simulink model "ME295B_Controller1Sim"  (R2018b)
settings: Solver=ode5  StartTime=0.0  StopTime=15  FixedStep=0.0001  RelTol=1e-3  EnableMultiTasking=on
values from neighbouring files (symbols this model uses):
  amp = [pi/4 pi/8 pi/5]    [ME295B_Controller1.m]
  freq = [f f*2 f*3]    [ME295B_Controller1.m]
  Ka = 10.*diag(ones(1,length(Phi)))    [ME295B_Controller1.m]
  Lambda = (p/2).*diag(ones(1,3))    [ME295B_Controller1.m]
  Phi_hat_max = (1+BoundsRatio)*Phi_hat_o    [ME295B_Controller1.m]
  Phi_hat_min = (1-BoundsRatio)*Phi_hat_o    [ME295B_Controller1.m]
  Phi_hat_o = Phi.*z'    [ME295B_Controller1.m]
settings Model: Creator=Alan  LastModifiedBy=adeli
settings DataIOCC: LimitDataPoints=on  SaveFormat=Array
settings OptimizationCC: LifeSpan=inf
settings DebuggingCC: SFUnexpectedBacktrackingDiag=warning  SFNoUnconditionalDefaultTransitionDiag=warning  SFExecutionAtInitializationDiag=none
settings HardwareCC: ProdBitPerPointer=32  ProdBitPerSizeT=32  ProdBitPerPtrDiffT=32  ProdLargestAtomicFloat=None  ProdIntDivRoundTo=Undefined  ProdEndianess=Unspecified  ProdWordSize=32  ProdHWDeviceType=32-bit Generic
settings ModelReferenceCC: PropagateSignalLabelsOutOfModel=off
settings SFSimCC: SimUseLocalCustomCode=off
settings RTWCC: RTWUseLocalCustomCode=off
settings CodeAppCC: StateflowObjectComments=on
settings GRTTargetCC: TargetLangStandard=C89/C90 (ANSI)  GeneratePreprocessorConditionals=Disable all
settings ConfigComp: CovMetricSettings=dw  CovHtmlReporting=on  CovSaveCumulativeToWorkspaceVar=on  CovSaveSingleToWorkspaceVar=on  CovExternalEMLEnable=off

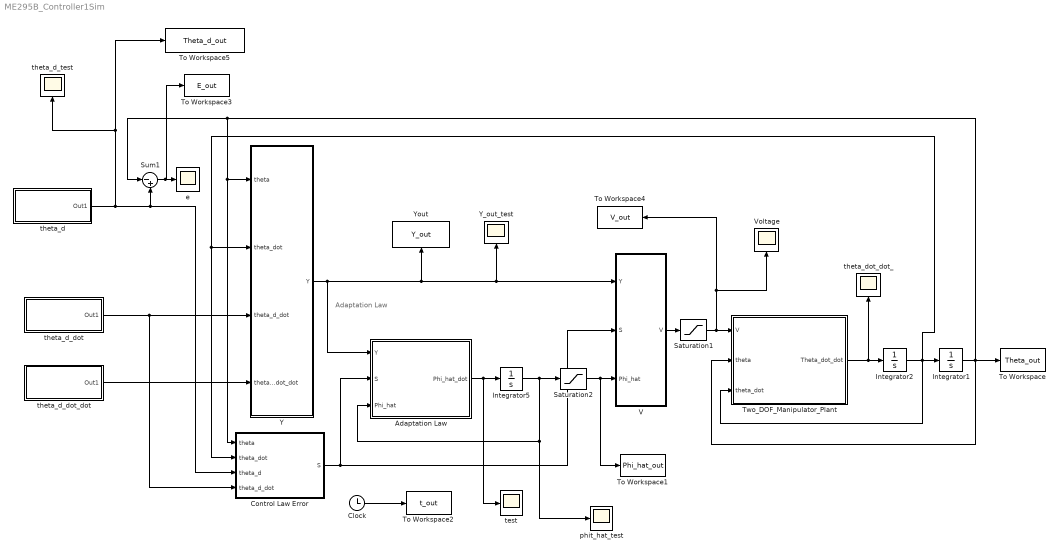
== system ME295B_Controller1Sim ==
  note: Adaptation Law
  Adaptation Law : MATLAB Function  TreatAsAtomicUnit=on
  Clock : Clock
  Control Law Error : MATLAB Function  TreatAsAtomicUnit=on
  Integrator1 : Integrator  InitialCondition=[0;0;0]
  Integrator2 : Integrator  InitialCondition=[0;0;0]
  Integrator5 : Integrator  InitialCondition=Phi_hat_o
  Saturation1 : Saturate  UpperLimit=[24, 24, 24]  LowerLimit=[-24, -24, -24]
  Saturation2 : Saturate  UpperLimit=1000000  LowerLimit=0
  Sum1 : Sum  Inputs=|-+
  To Workspace : ToWorkspace  VariableName=Theta_out  SampleTime=-1
  To Workspace1 : ToWorkspace  VariableName=Phi_hat_out  SampleTime=-1
  To Workspace2 : ToWorkspace  VariableName=t_out  SampleTime=-1
  To Workspace3 : ToWorkspace  VariableName=E_out  SampleTime=-1
  To Workspace4 : ToWorkspace  VariableName=V_out  SampleTime=-1
  To Workspace5 : ToWorkspace  VariableName=Theta_d_out  SampleTime=-1
  Two_DOF_Manipulator_Plant : MATLAB Function  TreatAsAtomicUnit=on
  V : MATLAB Function  TreatAsAtomicUnit=on
  Voltage : Scope
  Y : MATLAB Function  TreatAsAtomicUnit=on
  Y_out_test : Scope
  Yout : ToWorkspace  VariableName=Y_out  SampleTime=-1
  e : Scope
  "phit_hat_test " : Scope
  test : Scope
  theta_d : Subsystem
  theta_d_dot : Subsystem
  theta_d_dot_dot : Subsystem
  theta_d_test : Scope
  theta_dot_dot_ : Scope
  wires:
  theta_d_dot_dot/1(Out1) -> Y/4(theta_d_dot_dot)
  Integrator2/1 -> Integrator1/1, Two_DOF_Manipulator_Plant/3(theta_dot), Control Law Error/2(theta_dot), Y/2(theta_dot)
  Integrator1/1 -> To Workspace/1, Two_DOF_Manipulator_Plant/2(theta), Control Law Error/1(theta), Y/1(theta), Sum1/1
  Sum1/1 -> To Workspace3/1, e/1
  Y/1(Y) -> Yout/1, Y_out_test/1, V/1(Y), Adaptation Law/1(Y)
  Control Law Error/1(S) -> V/2(S), Adaptation Law/2(S)
  Adaptation Law/1(Phi_hat_dot) -> Integrator5/1, test/1
  Integrator5/1 -> Saturation2/1, Adaptation Law/3(Phi_hat), "phit_hat_test "/1
  Two_DOF_Manipulator_Plant/1(Theta_dot_dot) -> theta_dot_dot_/1, Integrator2/1
  Clock/1 -> To Workspace2/1
  theta_d_dot/1(Out1) -> Control Law Error/4(theta_d_dot), Y/3(theta_d_dot)
  Saturation2/1 -> To Workspace1/1, V/3(Phi_hat)
  V/1(V) -> Saturation1/1
  Saturation1/1 -> Voltage/1, To Workspace4/1, Two_DOF_Manipulator_Plant/1(V)
  theta_d/1(Out1) -> theta_d_test/1, To Workspace5/1, Control Law Error/3(theta_d), Sum1/2

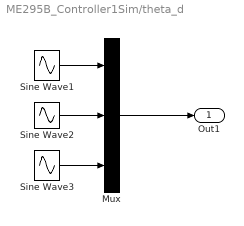
== system ME295B_Controller1Sim/theta_d ==
  Mux : Mux  Inputs=3
  Sine Wave1 : Sin  Amplitude=amp(1)  Frequency=freq(1)  SampleTime=0
  Sine Wave2 : Sin  Amplitude=amp(2)  Frequency=freq(2)  SampleTime=0
  Sine Wave3 : Sin  Amplitude=amp(1)  Frequency=freq(1)  SampleTime=0
  Out1 : Outport
  wires:
  Mux/1 -> Out1/1
  Sine Wave1/1 -> Mux/1
  Sine Wave2/1 -> Mux/2
  Sine Wave3/1 -> Mux/3

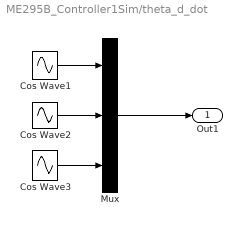
== system ME295B_Controller1Sim/theta_d_dot ==
  Cos Wave1 : Sin  Amplitude=freq(1)*amp(1)  Frequency=freq(1)  Phase=3.14/2  SampleTime=0
  Cos Wave2 : Sin  Amplitude=freq(2)*amp(2)  Frequency=freq(2)  Phase=3.14/2  SampleTime=0
  Cos Wave3 : Sin  Amplitude=freq(1)*amp(1)  Frequency=freq(1)  Phase=3.14/2  SampleTime=0
  Mux : Mux  Inputs=3
  Out1 : Outport
  wires:
  Mux/1 -> Out1/1
  Cos Wave1/1 -> Mux/1
  Cos Wave2/1 -> Mux/2
  Cos Wave3/1 -> Mux/3

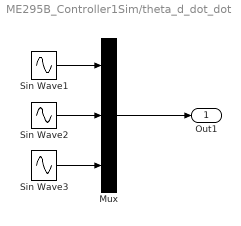
== system ME295B_Controller1Sim/theta_d_dot_dot ==
  Mux : Mux  Inputs=3
  Sin Wave1 : Sin  Amplitude=-freq(1)*freq(1)*amp(1)  Frequency=freq(1)  Phase=3.14/2  SampleTime=0
  Sin Wave2 : Sin  Amplitude=-freq(2)*freq(2)*amp(2)  Frequency=freq(2)  Phase=3.14/2  SampleTime=0
  Sin Wave3 : Sin  Amplitude=-freq(1)*freq(1)*amp(1)  Frequency=freq(1)  Phase=3.14/2  SampleTime=0
  Out1 : Outport
  wires:
  Mux/1 -> Out1/1
  Sin Wave1/1 -> Mux/1
  Sin Wave2/1 -> Mux/2
  Sin Wave3/1 -> Mux/3

== matlab function ME295B_Controller1Sim/V ==
  data: Eta parameter; V output; Y input; S input; Phi_hat input
function V = fcn(Eta, Y, S, Phi_hat)

V = (Y*Phi_hat) + Eta*S;

== matlab function ME295B_Controller1Sim/Y ==
  data: Lambda parameter; Y output; theta input; theta_dot input; theta_d_dot input; theta_d_dot_dot input; Phi_hat_o parameter
function Y = fcn(Lambda, theta, theta_dot,...
    theta_d_dot, theta_d_dot_dot, Phi_hat_o)

%errors and lambdas
e_dot1 = theta_d_dot(1,1)-theta_dot(1,1);
e_dot2 = theta_d_dot(2,1)-theta_dot(2,1);
e_dot3 = theta_d_dot(3,1)-theta_dot(3,1);

lambda1= Lambda(1,1);
lambda2 = Lambda(2,2);
lambda3 = Lambda(3,3);

theta_dot_dot1 = theta_d_dot_dot(1,1)+(lambda1*e_dot1);
theta_dot_dot2 = theta_d_dot_dot(2,1)+(lambda2*e_dot2);
theta_dot_dot3 = theta_d_dot_dot(3,1)+(lambda3*e_dot3);

%beta2 divided by beta1
k2_k1 = Phi_hat_o(2)/Phi_hat_o(1);
k3_k1 = Phi_hat_o(3)/Phi_hat_o(1);
k3_k2 = Phi_hat_o(3)/Phi_hat_o(2);

%first linkage
y11 = 2*( theta_dot_dot1*cos(theta(2,1)*cos(theta(2,1)+theta(3,1))) -...
    (theta_dot(1,1)*theta_dot(3,1)*cos(theta(2,1))*sin(theta(2,1)+theta(3,1))) -...
    (theta_dot(1,1)*theta_dot(2,1)*sin( (2*theta(2,1)) +theta(3,1))) );
y12=0;
y13=0;
y14 = 0;
y15 = (theta_dot_dot1)*(cos(theta(2,1))^2 ) +...
    -(2*theta_dot(1,1)*theta_dot(2,1)*sin(2*theta(2,1)));
y16 = (theta_dot_dot1)*(cos(theta(2,1)+theta(3,1)))^2 +...
    -2*theta_dot(1,1)*theta_dot(3,1)*cos(theta(2,1)+theta(3,1))*sin(theta(2,1)+theta(3,1)) +...
    -2*theta_dot(1,1)*theta_dot(2,1)*sin(2*(theta_dot(2,1)+theta(3,1)));
y17 = (sin(theta(2,1))^2)+...
    (2*theta_dot(1,1)*theta_dot(2,1)*sin(2*theta(2,1)));
y18 = (theta_dot_dot1)*(sin(theta(2,1)+theta(3,1))^2)+...
    2*theta_dot(1,1)*theta_dot(3,1)*cos(theta(2,1)+theta(3,1))*sin(theta(2,1)+theta(3,1)) +...
    2*theta_dot(1,1)*theta_dot(2,1)*sin(2*(theta_dot(2,1)+theta(3,1)));
y19 = theta_dot_dot1;
y110 = 0;
y111 = 0;
y112 = 0;
y113 = 0;
y114 = theta_dot(1,1);
y115 = 0;
y116 = 0;
%second linkage
y21 = 0;
y22 =2*theta_dot_dot2 +...
    theta_dot_dot3*cos(theta(3,1)) - ...
    theta_dot(3,1)*(theta_dot(2,1)+theta_dot(3,1)) -...
    (theta_dot(2,1)*theta_dot(3,1)*sin(theta(3,1))) +...
    (theta_dot(1,1)^2)*sin( (2*theta(2,1)) +theta(3,1));
y23 = 0;
y24 = -cos(theta(2,1))+...
    cos(theta(2,1)+theta(3,1));
y25 = k2_k1*(0.5*theta_dot(1,1)^2)*sin(2*theta(2,1));
y26 = k2_k1*(0.5*(theta_dot(1,1)^2)*sin(2*(theta(2,1)+theta(3,1))) );
y27 = k2_k1*(-0.5*theta_dot(1,1)^2)*sin(2*theta(2,1));
y28 = k2_k1*(-0.5*(theta_dot(1,1)^2)*sin(2*(theta(2,1)+theta(3,1))) );
y29 = 0;
y210 = sin(theta(2,1));
y211 =sin(theta(2,1)+theta(3,1));
y212= theta_dot_dot3;
y213=theta_dot_dot2;
y214=0;
y215=theta_dot(2,1);
y216=0;
%3rd linkage
y31 = 0;
y32 =0;
y33 = (theta_dot(1,1)^2)*cos(theta(2,1))*sin(theta(2,1)+theta(3,1)) +...
    theta_dot_dot2*cos(theta(3,1)) +...
    sin(theta(3,1));
y34 = 0;
y35 = 0;
y36 = k3_k1*(theta_dot(1,1)^2)*cos(theta(2,1)+theta(3,1))*sin(theta(2,1)+theta(3,1)) ;
y37 = 0;
y38 = k3_k1*(-theta_dot(1,1)^2)*cos(theta(2,1)+theta(3,1))*sin(theta(2,1)+theta(3,1)) ;
y39 = 0;
y310 = 0;
y311 =k3_k2*sin(theta(2,1)+theta(3,1));
y312= k3_k2*(theta_dot_dot2+theta_dot_dot3);
y313=0;
y314=0;
y315=0;
y316=theta_dot(3,1);

Y = [y11 y12 y13 y14 y15 y16 y17 y18 y19 y110 y111 y112 y113 y114 y115 y116 ;
    y21 y22 y23 y24 y25 y26 y27 y28 y29 y210 y211 y212 y213 y214 y215 y216;
    y31 y32 y33 y34 y35 y36 y37 y38 y39 y310 y311 y312 y313 y314 y315 y316];

== matlab function ME295B_Controller1Sim/Adaptation Law ==
  data: Phi_hat_max parameter; Phi_hat_dot output; Phi_hat_min parameter; Ka parameter; Y input; S input; Phi_hat input
function Phi_hat_dot = fcn(Phi_hat_max, Phi_hat_min, Ka, Y, S, Phi_hat)


%matrix multiplication of Y transpose and S
YTS = transpose(Y)*S;

%if any of the adaptive parameters exceed bounds then set them equal to 0
%this derives from the "proj" function
for i=1:length(Phi_hat)
    %phi matrices with lower/upper bounds
    if(YTS(i)>0 && Phi_hat(i)>=Phi_hat_max(i))
        YTS(i) = 0;
    elseif(YTS(i)<0 && Phi_hat(i)<= Phi_hat_min(i))
        YTS(i) = 0;
    end
end


Phi_hat_dot = Ka*YTS;

== matlab function ME295B_Controller1Sim/Control Law Error ==
  data: Lambda parameter; S output; theta input; theta_dot input; theta_d input; theta_d_dot input
function S = fcn(Lambda, theta, theta_dot, theta_d, theta_d_dot)
lambda1 = Lambda(1,1);
lambda2 = Lambda(2,2);
lambda3 = Lambda(3,3);

e1 = theta_d(1)-theta(1);
e_dot1 = theta_d_dot(1) - theta_dot(1);
e2 = theta_d(2)-theta(2);
e_dot2 = theta_d_dot(2) - theta_dot(2);
e3 = theta_d(3)-theta(3);
e_dot3 = theta_d_dot(3) - theta_dot(3);

s1 = e_dot1 + lambda1*e1;
s2 = e_dot2 + lambda2*e2;
s3 = e_dot3 + lambda3*e3;

S = [s1; s2; s3];

== matlab function ME295B_Controller1Sim/Two_DOF_Manipulator_Plant ==
  data: Phi parameter; Theta_dot_dot output; V input; theta input; theta_dot input
function Theta_dot_dot = fcn(Phi, V, theta, theta_dot)

K1 = Phi(1);
K2 = Phi(2);
K3 = Phi(3);
K4 = Phi(4);
K5 = Phi(5);
K6 = Phi(6);
K7 = Phi(7);
K8 = Phi(8);
K9 = Phi(9);
K10 = Phi(10);
K11 = Phi(11);
K12 = Phi(12);
K13 = Phi(13);
K14 = Phi(14);
K15 = Phi(15);
K16 = Phi(16);

M11 =K5*(cos(theta(2,1))^2)+...
    (2*K1*cos(theta(2,1))*cos(theta(2,1)+theta(3,1)))+...
    K6*(cos(theta(2,1)+theta(3,1)))^2 +...
    K7*(sin(theta(2,1))^2) +...
    K8*(sin(theta(2,1)+theta(3,1))^2) +...
    K9;
M12=0;
M13=0;
M21=0;
M22= 2*K2*cos(theta(3,1)) + K13;
M23= K2*cos(theta(3,1))+K12;
M31=0;
M32=K3*cos(theta(3,1)) + K3*K12;
M33=K3/K2*K12;

C11 = (-K1*theta_dot(3,1)*cos(theta(2,1))*sin(theta(2,1)+theta(3,1)))-...
    ( (K6-K8)*theta_dot(3,1)*cos(theta(2,1)+theta(3,1))*sin(theta(2,1)+theta(3,1)) ) -...
    ( 0.5*(K6-K8)*theta_dot(2,1)*sin(2*(theta(2,1)+theta(3,1))) ) -...
    K1*theta_dot(2,1)*sin((2*theta(2,1))+theta(3,1)) -...
    (0.5*(K5-K7)*theta_dot(2,1)*sin(2*theta(2,1))) +...
    K14;
C12= (-0.5*(K6-K8)*theta_dot(1,1)*sin(2*(theta(2,1)+theta(3,1))) ) -...
    (K1*theta_dot(1,1)*sin((2*theta(2,1))+theta(3,1)) )-...
    (0.5*(K5-K7)*theta_dot(1,1)*sin(2*theta(2,1)));
C13=-(K1*theta_dot(1,1)*cos(theta(2,1))*sin(theta(2,1) + theta(3,1))) -...
    ((K6-K8)*theta_dot(1,1)*cos(theta(2,1)+theta(3,1))*sin(theta(2,1)+theta(3,1)));
C21= (0.5*(K2/K1)*(K6-K8)*theta_dot(1,1)*sin(2*(theta(2,1)+theta(3,1))) )+...
    K2*theta_dot(1,1)*sin( (2*theta(2,1)) +theta(3,1)) +...
    (0.5*(K2/K1)*(K5-K7)*sin(2*theta(2,1))*theta_dot(1,1));
C22= (-K2*theta_dot(3,1)*sin(theta(3,1)))+K15;
C23= -K2*(theta_dot(2,1)+theta_dot(3,1))*sin(theta(3,1));
C31= K3*theta_dot(1,1)*cos(theta(2,1))*sin(theta(2,1)+theta(3,1)) + ...
    (K3/K1)*(K6-K8)*theta_dot(1,1)*cos(theta(2,1)+theta(3,1))*sin(theta(2,1)+theta(3,1));
C32=K3*theta_dot(2,1)*sin(theta(3,1));
C33=K16;

N1 = 0;
N2 = -K4*cos(theta(2,1)) +...
    K4*cos(theta(2,1)+theta(3,1))+...
    K10*sin(theta(2,1))+...
    K11*sin(theta(2,1)+theta(3,1));
N3 = ( (K3/K2)*K4*cos(theta(2,1)+theta(3,1)) ) +...
    ((K3/K2)*K11*cos(theta(2,1)+theta(3,1)));

M = [M11 M12 M13; M21 M22 M23; M31 M32 M33];
C = [ C11 C12 C13; C21 C22 C23; C31 C32 C33];
N = [N1; N2; N3];

Theta_dot_dot = inv(M)*(V-(C*theta_dot)-N);
